simulink model "Dynamic_Formation"  (R2014a)
settings: Solver=ode45  StartTime=0.0  StopTime=800  RelTol=1e-3
settings Model: Creator=asus  LastModifiedBy=asus

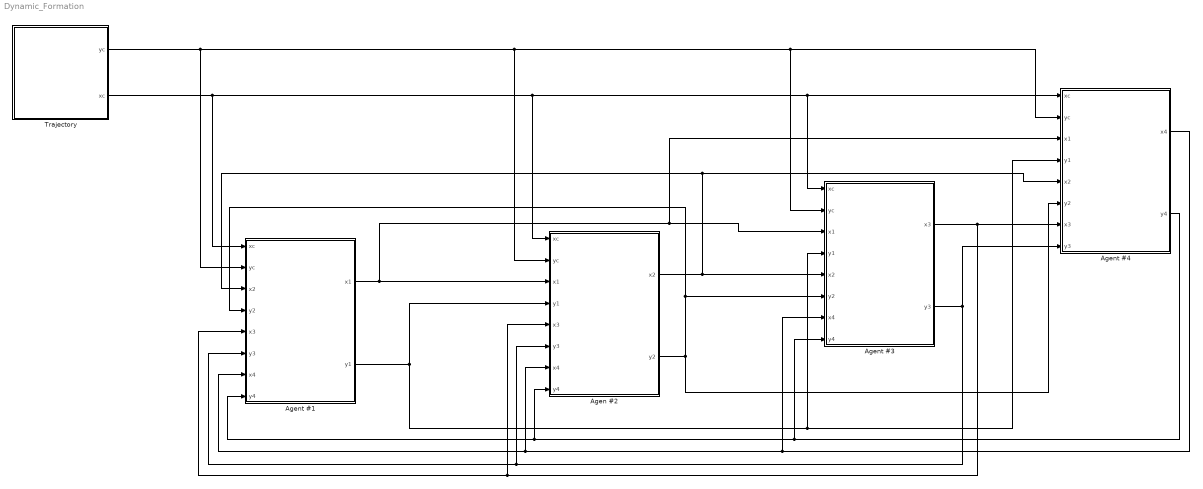
== system Dynamic_Formation ==
  "Agen #2 " : Subsystem
  "Agent #1 " : Subsystem
  Agent #3 : Subsystem
  Agent #4 : Subsystem
  Trajectory : Subsystem
  wires:
  "Agent #1 "/1(x1) -> Agent #4/3(x1), Agent #3/3(x1), "Agen #2 "/3(x1)
  "Agent #1 "/2(y1) -> "Agen #2 "/4(y1), Agent #3/4(y1), Agent #4/4(y1)
  Agent #3/1(x3) -> "Agent #1 "/5(x3), "Agen #2 "/5(x3), Agent #4/7(x3)
  Agent #3/2(y3) -> "Agent #1 "/6(y3), "Agen #2 "/6(y3), Agent #4/8(y3)
  Trajectory/2(xc) -> "Agen #2 "/1(xc), Agent #3/1(xc), Agent #4/1(xc), "Agent #1 "/1(xc)
  Trajectory/1(yc) -> "Agen #2 "/2(yc), Agent #3/2(yc), Agent #4/2(yc), "Agent #1 "/2(yc)
  Agent #4/2(y4) -> "Agent #1 "/8(y4), "Agen #2 "/8(y4), Agent #3/8(y4)
  Agent #4/1(x4) -> "Agent #1 "/7(x4), "Agen #2 "/7(x4), Agent #3/7(x4)
  "Agen #2 "/1(x2) -> "Agent #1 "/3(x2), Agent #4/5(x2), Agent #3/5(x2)
  "Agen #2 "/2(y2) -> Agent #3/6(y2), "Agent #1 "/4(y2), Agent #4/6(y2)

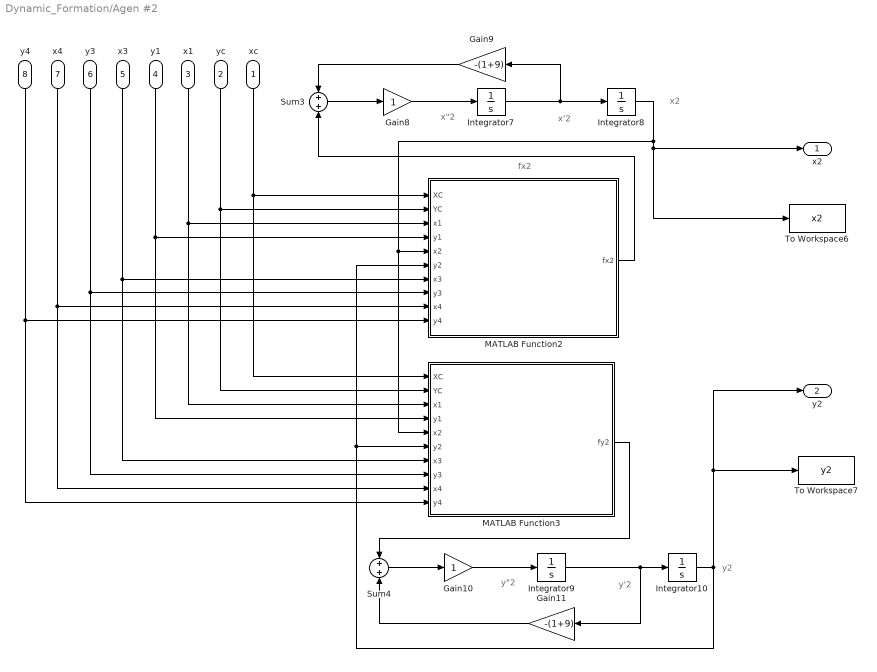
== system Dynamic_Formation/Agen #2  ==
  note: x2
  note: x'2
  note: x"2
  note: fx2
  note: y2
  note: y'2
  note: y"2
  xc : Inport
  yc : Inport  Port=2
  x1 : Inport  Port=3
  y1 : Inport  Port=4
  x3 : Inport  Port=5
  y3 : Inport  Port=6
  x4 : Inport  Port=7
  y4 : Inport  Port=8
  Gain10 : Gain
  Gain11 : Gain  Gain=-(1+9)
  Gain8 : Gain
  Gain9 : Gain  Gain=-(1+9)
  Integrator10 : Integrator  InitialCondition=6
  Integrator7 : Integrator
  Integrator8 : Integrator  InitialCondition=3
  Integrator9 : Integrator
  MATLAB Function2 : MATLAB Function  TreatAsAtomicUnit=on
  MATLAB Function3 : MATLAB Function  TreatAsAtomicUnit=on
  Sum3 : Sum  Inputs=+|+
  Sum4 : Sum  Inputs=+|+
  To Workspace6 : ToWorkspace  VariableName=x2  SampleTime=0.01
  To Workspace7 : ToWorkspace  VariableName=y2  SampleTime=0.01
  x2 : Outport
  y2 : Outport  Port=2
  wires:
  Sum3/1 -> Gain8/1
  Gain8/1 -> Integrator7/1
  Integrator7/1 -> Gain9/1, Integrator8/1
  Gain9/1 -> Sum3/1
  Integrator8/1 -> To Workspace6/1, x2/1, MATLAB Function3/5(x2), MATLAB Function2/5(x2)
  MATLAB Function2/1(fx2) -> Sum3/2
  Sum4/1 -> Gain10/1
  Gain10/1 -> Integrator9/1
  Integrator9/1 -> Gain11/1, Integrator10/1
  Gain11/1 -> Sum4/2
  MATLAB Function3/1(fy2) -> Sum4/1
  Integrator10/1 -> y2/1, To Workspace7/1, MATLAB Function2/6(y2), MATLAB Function3/6(y2)
  xc/1 -> MATLAB Function2/1(XC), MATLAB Function3/1(XC)
  yc/1 -> MATLAB Function2/2(YC), MATLAB Function3/2(YC)
  y1/1 -> MATLAB Function2/4(y1), MATLAB Function3/4(y1)
  x1/1 -> MATLAB Function2/3(x1), MATLAB Function3/3(x1)
  x3/1 -> MATLAB Function2/7(x3), MATLAB Function3/7(x3)
  y3/1 -> MATLAB Function2/8(y3), MATLAB Function3/8(y3)
  x4/1 -> MATLAB Function2/9(x4), MATLAB Function3/9(x4)
  y4/1 -> MATLAB Function2/10(y4), MATLAB Function3/10(y4)

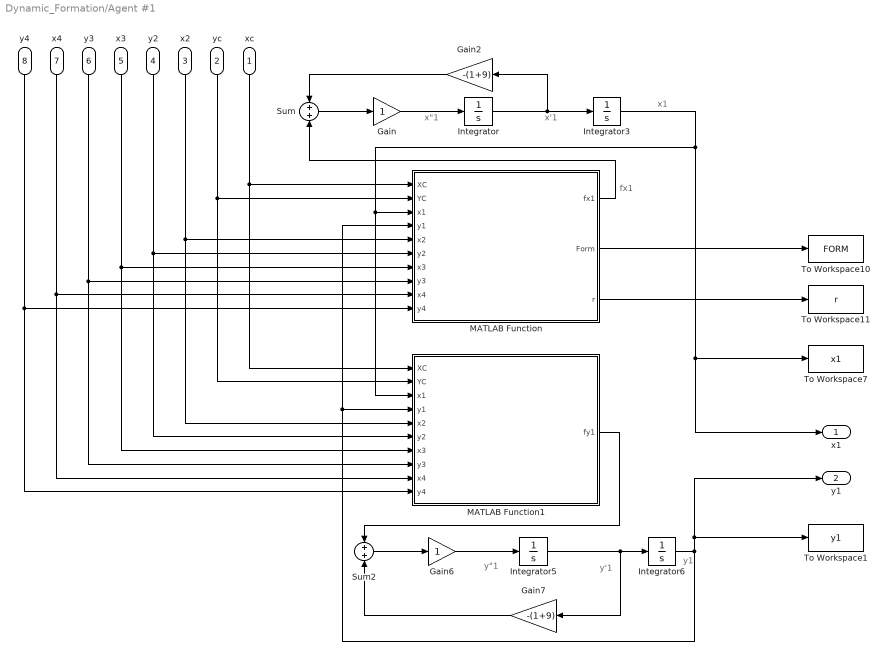
== system Dynamic_Formation/Agent #1  ==
  note: x1
  note: x'1
  note: x"1
  note: fx1
  note: y1
  note: y'1
  note: y"1
  xc : Inport
  yc : Inport  Port=2
  x2 : Inport  Port=3
  y2 : Inport  Port=4
  x3 : Inport  Port=5
  y3 : Inport  Port=6
  x4 : Inport  Port=7
  y4 : Inport  Port=8
  Gain : Gain
  Gain2 : Gain  Gain=-(1+9)
  Gain6 : Gain
  Gain7 : Gain  Gain=-(1+9)
  Integrator : Integrator
  Integrator3 : Integrator  InitialCondition=-1
  Integrator5 : Integrator
  Integrator6 : Integrator  InitialCondition=2
  MATLAB Function : MATLAB Function  TreatAsAtomicUnit=on
  MATLAB Function1 : MATLAB Function  TreatAsAtomicUnit=on
  Sum : Sum  Inputs=+|+
  Sum2 : Sum  Inputs=+|+
  To Workspace1 : ToWorkspace  VariableName=y1  SampleTime=0.01
  To Workspace10 : ToWorkspace  VariableName=FORM  SampleTime=0.01
  To Workspace11 : ToWorkspace  VariableName=r  SampleTime=1
  To Workspace7 : ToWorkspace  VariableName=x1  SampleTime=0.01
  x1 : Outport
  y1 : Outport  Port=2
  wires:
  Sum/1 -> Gain/1
  Gain/1 -> Integrator/1
  Integrator/1 -> Gain2/1, Integrator3/1
  Gain2/1 -> Sum/1
  Sum2/1 -> Gain6/1
  Gain6/1 -> Integrator5/1
  Integrator5/1 -> Gain7/1, Integrator6/1
  Gain7/1 -> Sum2/2
  MATLAB Function1/1(fy1) -> Sum2/1
  Integrator6/1 -> MATLAB Function/4(y1), MATLAB Function1/4(y1), To Workspace1/1, y1/1
  MATLAB Function/1(fx1) -> Sum/2
  MATLAB Function/2(Form) -> To Workspace10/1
  MATLAB Function/3(r) -> To Workspace11/1
  Integrator3/1 -> MATLAB Function1/3(x1), MATLAB Function/3(x1), To Workspace7/1, x1/1
  xc/1 -> MATLAB Function/1(XC), MATLAB Function1/1(XC)
  yc/1 -> MATLAB Function/2(YC), MATLAB Function1/2(YC)
  x2/1 -> MATLAB Function/5(x2), MATLAB Function1/5(x2)
  y2/1 -> MATLAB Function/6(y2), MATLAB Function1/6(y2)
  x3/1 -> MATLAB Function/7(x3), MATLAB Function1/7(x3)
  y3/1 -> MATLAB Function/8(y3), MATLAB Function1/8(y3)
  x4/1 -> MATLAB Function/9(x4), MATLAB Function1/9(x4)
  y4/1 -> MATLAB Function/10(y4), MATLAB Function1/10(y4)

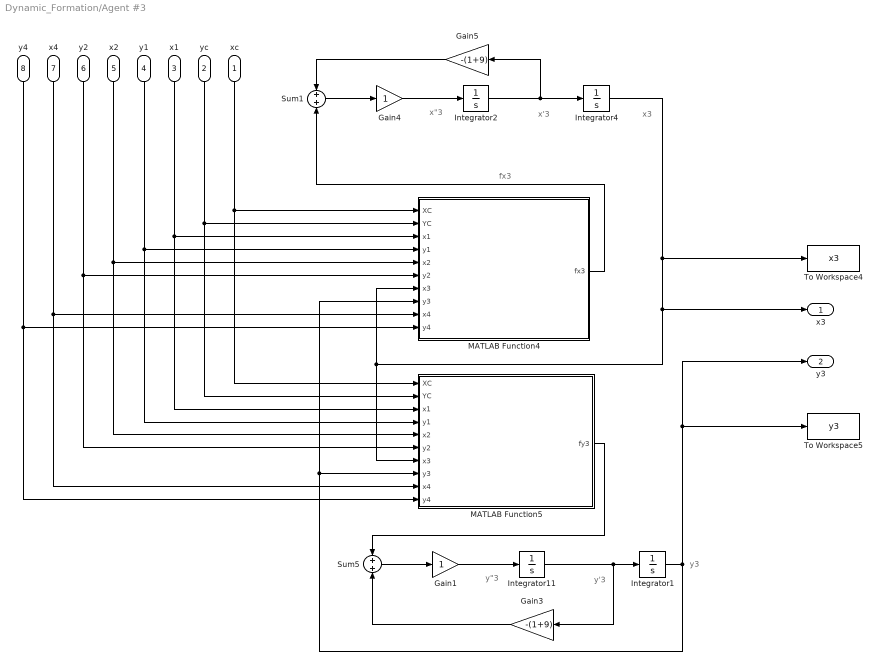
== system Dynamic_Formation/Agent #3 ==
  note: x3
  note: x'3
  note: x"3
  note: fx3
  note: y3
  note: y'3
  note: y"3
  xc : Inport
  yc : Inport  Port=2
  x1 : Inport  Port=3
  y1 : Inport  Port=4
  x2 : Inport  Port=5
  y2 : Inport  Port=6
  x4 : Inport  Port=7
  y4 : Inport  Port=8
  Gain1 : Gain
  Gain3 : Gain  Gain=-(1+9)
  Gain4 : Gain
  Gain5 : Gain  Gain=-(1+9)
  Integrator1 : Integrator  InitialCondition=-1
  Integrator11 : Integrator
  Integrator2 : Integrator
  Integrator4 : Integrator  InitialCondition=3
  MATLAB Function4 : MATLAB Function  TreatAsAtomicUnit=on
  MATLAB Function5 : MATLAB Function  TreatAsAtomicUnit=on
  Sum1 : Sum  Inputs=+|+
  Sum5 : Sum  Inputs=+|+
  To Workspace4 : ToWorkspace  VariableName=x3  SampleTime=0.01
  To Workspace5 : ToWorkspace  VariableName=y3  SampleTime=0.01
  x3 : Outport
  y3 : Outport  Port=2
  wires:
  Sum1/1 -> Gain4/1
  Gain4/1 -> Integrator2/1
  Integrator2/1 -> Gain5/1, Integrator4/1
  Gain5/1 -> Sum1/1
  MATLAB Function4/1(fx3) -> Sum1/2
  Sum5/1 -> Gain1/1
  Gain1/1 -> Integrator11/1
  Integrator11/1 -> Gain3/1, Integrator1/1
  Gain3/1 -> Sum5/2
  MATLAB Function5/1(fy3) -> Sum5/1
  Integrator1/1 -> MATLAB Function5/8(y3), MATLAB Function4/8(y3), To Workspace5/1, y3/1
  Integrator4/1 -> x3/1, MATLAB Function5/7(x3), MATLAB Function4/7(x3), To Workspace4/1
  xc/1 -> MATLAB Function4/1(XC), MATLAB Function5/1(XC)
  yc/1 -> MATLAB Function5/2(YC), MATLAB Function4/2(YC)
  x1/1 -> MATLAB Function4/3(x1), MATLAB Function5/3(x1)
  y1/1 -> MATLAB Function4/4(y1), MATLAB Function5/4(y1)
  x2/1 -> MATLAB Function4/5(x2), MATLAB Function5/5(x2)
  y2/1 -> MATLAB Function4/6(y2), MATLAB Function5/6(y2)
  x4/1 -> MATLAB Function4/9(x4), MATLAB Function5/9(x4)
  y4/1 -> MATLAB Function4/10(y4), MATLAB Function5/10(y4)

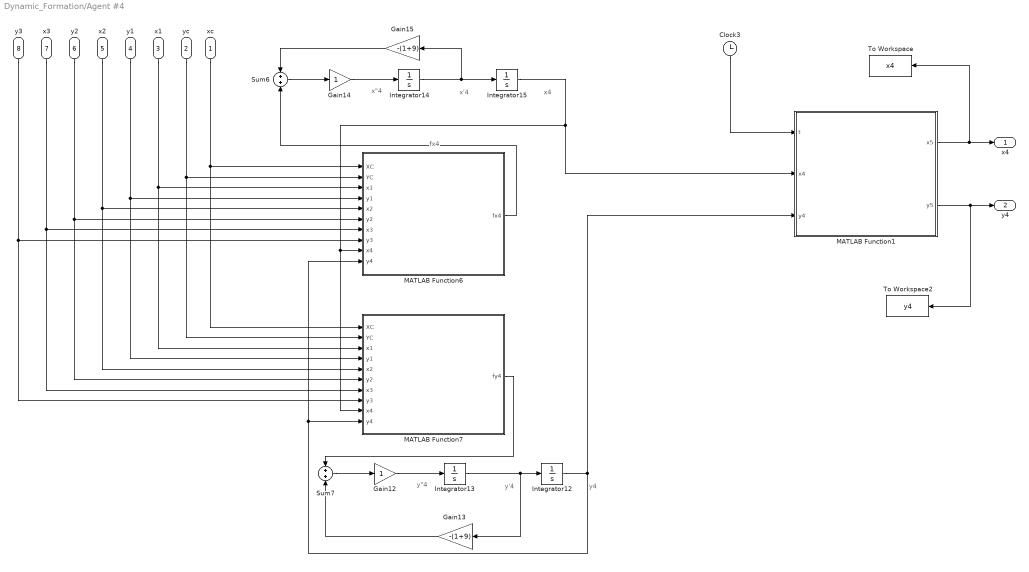
== system Dynamic_Formation/Agent #4 ==
  note: x4
  note: x'4
  note: x"4
  note: fx4
  note: y4
  note: y'4
  note: y"4
  xc : Inport
  yc : Inport  Port=2
  x1 : Inport  Port=3
  y1 : Inport  Port=4
  x2 : Inport  Port=5
  y2 : Inport  Port=6
  x3 : Inport  Port=7
  y3 : Inport  Port=8
  Clock3 : Clock
  Gain12 : Gain
  Gain13 : Gain  Gain=-(1+9)
  Gain14 : Gain
  Gain15 : Gain  Gain=-(1+9)
  Integrator12 : Integrator  InitialCondition=-4
  Integrator13 : Integrator
  Integrator14 : Integrator
  Integrator15 : Integrator  InitialCondition=-4
  MATLAB Function1 : MATLAB Function  TreatAsAtomicUnit=on
  MATLAB Function6 : MATLAB Function  TreatAsAtomicUnit=on
  MATLAB Function7 : MATLAB Function  TreatAsAtomicUnit=on
  Sum6 : Sum  Inputs=+|+
  Sum7 : Sum  Inputs=+|+
  To Workspace : ToWorkspace  VariableName=x4  SampleTime=0.01
  To Workspace2 : ToWorkspace  VariableName=y4  SampleTime=0.01
  x4 : Outport
  y4 : Outport  Port=2
  wires:
  Sum6/1 -> Gain14/1
  Gain14/1 -> Integrator14/1
  Integrator14/1 -> Gain15/1, Integrator15/1
  Gain15/1 -> Sum6/1
  Integrator15/1 -> MATLAB Function1/2(x4), MATLAB Function7/9(x4), MATLAB Function6/9(x4)
  MATLAB Function6/1(fx4) -> Sum6/2
  Sum7/1 -> Gain12/1
  Gain12/1 -> Integrator13/1
  Integrator13/1 -> Gain13/1, Integrator12/1
  Gain13/1 -> Sum7/2
  MATLAB Function7/1(fy4) -> Sum7/1
  Integrator12/1 -> MATLAB Function1/3(y4), MATLAB Function6/10(y4), MATLAB Function7/10(y4)
  Clock3/1 -> MATLAB Function1/1(t)
  xc/1 -> MATLAB Function6/1(XC), MATLAB Function7/1(XC)
  yc/1 -> MATLAB Function6/2(YC), MATLAB Function7/2(YC)
  x1/1 -> MATLAB Function6/3(x1), MATLAB Function7/3(x1)
  y1/1 -> MATLAB Function6/4(y1), MATLAB Function7/4(y1)
  x2/1 -> MATLAB Function6/5(x2), MATLAB Function7/5(x2)
  y2/1 -> MATLAB Function6/6(y2), MATLAB Function7/6(y2)
  x3/1 -> MATLAB Function6/7(x3), MATLAB Function7/7(x3)
  y3/1 -> MATLAB Function6/8(y3), MATLAB Function7/8(y3)
  MATLAB Function1/1(x5) -> To Workspace/1, x4/1
  MATLAB Function1/2(y5) -> To Workspace2/1, y4/1

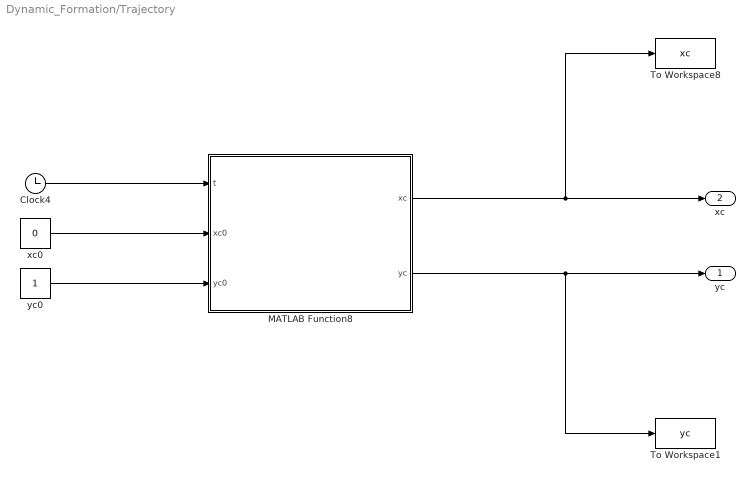
== system Dynamic_Formation/Trajectory ==
  Clock4 : Clock
  MATLAB Function8 : MATLAB Function  TreatAsAtomicUnit=on
  To Workspace1 : ToWorkspace  VariableName=yc  SampleTime=0.01
  To Workspace8 : ToWorkspace  VariableName=xc  SampleTime=0.01
  xc0 : Constant  Value=0
  yc0 : Constant
  yc : Outport
  xc : Outport  Port=2
  wires:
  xc0/1 -> MATLAB Function8/2(xc0)
  yc0/1 -> MATLAB Function8/3(yc0)
  Clock4/1 -> MATLAB Function8/1(t)
  MATLAB Function8/1(xc) -> To Workspace8/1, xc/1
  MATLAB Function8/2(yc) -> To Workspace1/1, yc/1

== matlab function Dynamic_Formation/Agent #1 /MATLAB Function1 ==
  data: XC input; YC input; fy1 output; x1 input; y1 input; x2 input; y2 input; x3 input; y3 input; x4 input; y4 input
function fy1 = fy1(XC,YC,x1,y1,x2,y2,x3,y3,x4,y4)
%#codegen
% Agent N#1
%xc = sin(t);
%yc = t;
%xc = XC;            % X-Center.
%yc = YC;            % Y-Center.
al = 3;             % Radius.
x = [x1 x2 x3 x4];      
y = [y1 y2 y3 y4];     
M = 1;              % Mass.
B = 1;              % Damper.
kd = 9;             % Overshoot Controlling Coefficient.
ks = 1;
q = 10;     % Charges.
kr = 0.15;
N = 4;              % Number od Agents.

r2 = zeros(N,N);
costet = zeros(N,N);
sintet = zeros(N,N);
Prx = zeros(N);
Pry = zeros(N);

fx = zeros(N);
fy = zeros(N);
Fx = zeros(N);
Fy = zeros(N);


d1 = sqrt(((x(1)-XC)^2)+((y(1)-YC)^2));
d2 = sqrt(((x(2)-XC)^2)+((y(2)-YC)^2));
d3 = sqrt(((x(3)-XC)^2)+((y(3)-YC)^2));
d4 = sqrt(((x(4)-XC)^2)+((y(4)-YC)^2));
    
m1 = d2-d1;
m2 = d3-d2;
m3 = d4-d3;
    
    if m1<0.00001
        if m2<0.00001
            if m3<0.00001
                Form = 1;
            else
                Form = 0;
            end
        else
            Form = 0;
        end
    else 
        Form = 0;
    end

    
%if Form==0
    xc = XC;            % X-Center.
    yc = YC;            % Y-Center.



for k=1:N
    
    for i=1:N
      Pr = 0;
      r2(k,i) = ((x(i)-x(k))^2)+((y(i)-y(k))^2);
    
      if i==k
         Prx(k) = Prx(k) + 0;
         Pry(k) = Pry(k) + 0;
      else
         costet(k,i) = (x(k)-x(i))/sqrt(r2(k,i));
         sintet(k,i) = (y(k)-y(i))/sqrt(r2(k,i));
         Prx(k) = Prx(k) + (q*q/r2(k,i))*costet(k,i);
         Pry(k) = Pry(k) + (q*q/r2(k,i))*sintet(k,i);
        
      end
    end

    Fx(k) = kr*Prx(k);
    Fy(k) = kr*Pry(k);
                        
    fx(k) = Fx(k)-ks*((x(k)-xc)*(((x(k)-xc)^2)+((y(k)-yc)^2)-al^2));
    fy(k) = Fy(k)-ks*((y(k)-yc)*(((x(k)-xc)^2)+((y(k)-yc)^2)-al^2));

end

fy1 = fy(1);

end

== matlab function Dynamic_Formation/Agent #1 /MATLAB Function ==
  data: XC input; YC input; fx1 output; x1 input; y1 input; x2 input; y2 input; x3 input; y3 input; x4 input; y4 input; Form output; r output
function [fx1,Form,r] = fx1(XC,YC,x1,y1,x2,y2,x3,y3,x4,y4)
%#codegen
% Agent N#1

xc = XC;            % X-Center.
yc = YC;            % Y-Center.
%xc = 0;            % X-Center.
%yc = 0;            % Y-Center.
al = 3;             % Radius.
x = [x1 x2 x3 x4];  % x vector.    
y = [y1 y2 y3 y4];  % y vector.   
M = 1;              % Mass.
B = 1;              % Damper.
kd = 9;             % Overshoot Controlling Coefficient.
ks = 1;
q = 10;             % Charges.
kr = 0.15;
N = 4;              % Number od Agents.
H = 0;

r2 = zeros(N,N);
costet = zeros(N,N);
sintet = zeros(N,N);
Prx = zeros(N);
Pry = zeros(N);
fx = zeros(N);
fy = zeros(N);
Fx = zeros(N);
Fy = zeros(N);

d1 = sqrt(((x(1)-XC)^2)+((y(1)-YC)^2));
d2 = sqrt(((x(2)-XC)^2)+((y(2)-YC)^2));
d3 = sqrt(((x(3)-XC)^2)+((y(3)-YC)^2));
d4 = sqrt(((x(4)-XC)^2)+((y(4)-YC)^2));

m1 = d2-d1;
m2 = d3-d2;
m3 = d4-d3;
    
    if m1<0.00001
        if m2<0.00001
            if m3<0.00001
                Form = 1;
            else
                Form = 0;
            end
        else
            Form = 0;
        end
    else 
        Form = 0;
    end


    
    for k=1:N
    
        for i=1:N
            Pr = 0;
            r2(k,i) = ((x(i)-x(k))^2)+((y(i)-y(k))^2);
    
         if i==k
             Prx(k) = Prx(k) + 0;
            Pry(k) = Pry(k) + 0;
         else
            costet(k,i) = (x(k)-x(i))/sqrt(r2(k,i));
            sintet(k,i) = (y(k)-y(i))/sqrt(r2(k,i));
            Prx(k) = Prx(k) + (q*q/r2(k,i))*costet(k,i);
            Pry(k) = Pry(k) + (q*q/r2(k,i))*sintet(k,i);
        
         end
        end

     Fx(k) = kr*Prx(k);
     Fy(k) = kr*Pry(k);
                        
     fx(k) = Fx(k)-ks*((x(k)-xc)*(((x(k)-xc)^2)+((y(k)-yc)^2)-al^2));
     fy(k) = Fy(k)-ks*((y(k)-yc)*(((x(k)-xc)^2)+((y(k)-yc)^2)-al^2));

    end

    fx1 = fx(1);
    r=r2;
    

   
    
    
    
    
    
    
    
    
    
    
    


end

== matlab function Dynamic_Formation/Agen #2 /MATLAB Function2 ==
  data: XC input; YC input; fx2 output; x1 input; y1 input; x2 input; y2 input; x3 input; y3 input; x4 input; y4 input
function fx2 = fx2(XC,YC,x1,y1,x2,y2,x3,y3,x4,y4)
%#codegen
% Agent N#1
%xc = XC;            % X-Center.
%yc = YC;            % Y-Center.
%xc = 0;             % X-Center.
%yc = 0;             % Y-Center.
al = 3;             % Radius.
x = [x1 x2 x3 x4];      
y = [y1 y2 y3 y4];     
M = 1;              % Mass.
B = 1;              % Damper.
kd = 9;             % Overshoot Controlling Coefficient.
ks = 1;
q = 10;     % Charges.
kr = 0.15;
N = 4;              % Number od Agents.

r2 = zeros(N,N);
costet = zeros(N,N);
sintet = zeros(N,N);
Prx = zeros(N);
Pry = zeros(N);

fx = zeros(N);
fy = zeros(N);
Fx = zeros(N);
Fy = zeros(N);

d1 = sqrt(((x(1)-XC)^2)+((y(1)-YC)^2));
d2 = sqrt(((x(2)-XC)^2)+((y(2)-YC)^2));
d3 = sqrt(((x(3)-XC)^2)+((y(3)-YC)^2));
d4 = sqrt(((x(4)-XC)^2)+((y(4)-YC)^2));
    
m1 = d2-d1;
m2 = d3-d2;
m3 = d4-d3;
    
    if m1<0.00001
        if m2<0.00001
            if m3<0.00001
                Form = 1;
            else
                Form = 0;
            end
        else
            Form = 0;
        end
    else 
        Form = 0;
    end

    
    xc = XC;            % X-Center.
    yc = YC;            % Y-Center.




for k=1:N
    
    for i=1:N
      Pr = 0;
      r2(k,i) = ((x(i)-x(k))^2)+((y(i)-y(k))^2);
    
      if i==k
         Prx(k) = Prx(k) + 0;
         Pry(k) = Pry(k) + 0;
      else
         costet(k,i) = (x(k)-x(i))/sqrt(r2(k,i));
         sintet(k,i) = (y(k)-y(i))/sqrt(r2(k,i));
         Prx(k) = Prx(k) + (q*q/r2(k,i))*costet(k,i);
         Pry(k) = Pry(k) + (q*q/r2(k,i))*sintet(k,i);
        
      end
    end

    Fx(k) = kr*Prx(k);
    Fy(k) = kr*Pry(k);
                        
    fx(k) = Fx(k)-ks*((x(k)-xc)*(((x(k)-xc)^2)+((y(k)-yc)^2)-al^2));
    fy(k) = Fy(k)-ks*((y(k)-yc)*(((x(k)-xc)^2)+((y(k)-yc)^2)-al^2));

end

fx2 = fx(2);


end

== matlab function Dynamic_Formation/Agen #2 /MATLAB Function3 ==
  data: XC input; YC input; fy2 output; x1 input; y1 input; x2 input; y2 input; x3 input; y3 input; x4 input; y4 input
function fy2 = fy2(XC,YC,x1,y1,x2,y2,x3,y3,x4,y4)
%#codegen
% Agent N#1
%yc = YC;            % Y-Center.
al = 3;             % Radius.
x = [x1 x2 x3 x4];      
y = [y1 y2 y3 y4];     
M = 1;              % Mass.
B = 1;              % Damper.
kd = 9;             % Overshoot Controlling Coefficient.
ks = 1;
q = 10;     % Charges.
kr = 0.15;
N = 4;              % Number od Agents.

r2 = zeros(N,N);
costet = zeros(N,N);
sintet = zeros(N,N);
Prx = zeros(N);
Pry = zeros(N);

fx = zeros(N);
fy = zeros(N);
Fx = zeros(N);
Fy = zeros(N);

d1 = sqrt(((x(1)-XC)^2)+((y(1)-YC)^2));
d2 = sqrt(((x(2)-XC)^2)+((y(2)-YC)^2));
d3 = sqrt(((x(3)-XC)^2)+((y(3)-YC)^2));
d4 = sqrt(((x(4)-XC)^2)+((y(4)-YC)^2));
    
m1 = d2-d1;
m2 = d3-d2;
m3 = d4-d3;
    
    if m1<0.00001
        if m2<0.00001
            if m3<0.00001
                Form = 1;
            else
                Form = 0;
            end
        else
            Form = 0;
        end
    else 
        Form = 0;
    end


    
    xc = XC;            % X-Center.
    yc = YC;            % Y-Center.




for k=1:N
    
    for i=1:N
      Pr = 0;
      r2(k,i) = ((x(i)-x(k))^2)+((y(i)-y(k))^2);
    
      if i==k
         Prx(k) = Prx(k) + 0;
         Pry(k) = Pry(k) + 0;
      else
         costet(k,i) = (x(k)-x(i))/sqrt(r2(k,i));
         sintet(k,i) = (y(k)-y(i))/sqrt(r2(k,i));
         Prx(k) = Prx(k) + (q*q/r2(k,i))*costet(k,i);
         Pry(k) = Pry(k) + (q*q/r2(k,i))*sintet(k,i);
        
      end
    end

    Fx(k) = kr*Prx(k);
    Fy(k) = kr*Pry(k);
                        
    fx(k) = Fx(k)-ks*((x(k)-xc)*(((x(k)-xc)^2)+((y(k)-yc)^2)-al^2));
    fy(k) = Fy(k)-ks*((y(k)-yc)*(((x(k)-xc)^2)+((y(k)-yc)^2)-al^2));

end

fy2 = fy(2);


end

== matlab function Dynamic_Formation/Agent #3/MATLAB Function4 ==
  data: XC input; YC input; fx3 output; x1 input; y1 input; x2 input; y2 input; x3 input; y3 input; x4 input; y4 input
function fx3 = fx3(XC,YC,x1,y1,x2,y2,x3,y3,x4,y4)
%#codegen
% Agent N#1
al = 3;             % Radius.
x = [x1 x2 x3 x4];      
y = [y1 y2 y3 y4];     
M = 1;              % Mass.
B = 1;              % Damper.
kd = 9;             % Overshoot Controlling Coefficient.
ks = 1;
q = 10;     % Charges.
kr = 0.15;
N = 4;              % Number od Agents.

r2 = zeros(N,N);
costet = zeros(N,N);
sintet = zeros(N,N);
Prx = zeros(N);
Pry = zeros(N);

fx = zeros(N);
fy = zeros(N);
Fx = zeros(N);
Fy = zeros(N);


Form = 0;
d1 = sqrt(((x(1)-XC)^2)+((y(1)-YC)^2));
d2 = sqrt(((x(2)-XC)^2)+((y(2)-YC)^2));
d3 = sqrt(((x(3)-XC)^2)+((y(3)-YC)^2));
d4 = sqrt(((x(4)-XC)^2)+((y(4)-YC)^2));
    
m1 = d2-d1;
m2 = d3-d2;
m3 = d4-d3;
    
    if m1<0.00001
        if m2<0.00001
            if m3<0.00001
                Form = 1;
            end
        end
    end

    
    xc = XC;            % X-Center.
    yc = YC;            % Y-Center.




for k=1:N
    
    for i=1:N
      Pr = 0;
      r2(k,i) = ((x(i)-x(k))^2)+((y(i)-y(k))^2);
    
      if i==k
         Prx(k) = Prx(k) + 0;
         Pry(k) = Pry(k) + 0;
      else
         costet(k,i) = (x(k)-x(i))/sqrt(r2(k,i));
         sintet(k,i) = (y(k)-y(i))/sqrt(r2(k,i));
         Prx(k) = Prx(k) + (q*q/r2(k,i))*costet(k,i);
         Pry(k) = Pry(k) + (q*q/r2(k,i))*sintet(k,i);
        
      end
    end

    Fx(k) = kr*Prx(k);
    Fy(k) = kr*Pry(k);
                        
    fx(k) = Fx(k)-ks*((x(k)-xc)*(((x(k)-xc)^2)+((y(k)-yc)^2)-al^2));
    fy(k) = Fy(k)-ks*((y(k)-yc)*(((x(k)-xc)^2)+((y(k)-yc)^2)-al^2));

end

fx3 = fx(3);


end

== matlab function Dynamic_Formation/Agent #3/MATLAB Function5 ==
  data: XC input; YC input; fy3 output; x1 input; y1 input; x2 input; y2 input; x3 input; y3 input; x4 input; y4 input
function fy3 = fy3(XC,YC,x1,y1,x2,y2,x3,y3,x4,y4)
%#codegen
al = 3;             % Radius.
x = [x1 x2 x3 x4];      
y = [y1 y2 y3 y4];     
M = 1;              % Mass.
B = 1;              % Damper.
kd = 9;             % Overshoot Controlling Coefficient.
ks = 1;
q = 10;     % Charges.
kr = 0.15;
N = 4;              % Number od Agents.

r2 = zeros(N,N);
costet = zeros(N,N);
sintet = zeros(N,N);
Prx = zeros(N);
Pry = zeros(N);

fx = zeros(N);
fy = zeros(N);
Fx = zeros(N);
Fy = zeros(N);

Form = 0;
d1 = sqrt(((x(1)-XC)^2)+((y(1)-YC)^2));
d2 = sqrt(((x(2)-XC)^2)+((y(2)-YC)^2));
d3 = sqrt(((x(3)-XC)^2)+((y(3)-YC)^2));
d4 = sqrt(((x(4)-XC)^2)+((y(4)-YC)^2));
    
m1 = d2-d1;
m2 = d3-d2;
m3 = d4-d3;
    
    if m1<0.00001
        if m2<0.00001
            if m3<0.00001
                Form = 1;
            end
        end
    end

    
%if Form==0
    xc = XC;            % X-Center.
    yc = YC;            % Y-Center.



for k=1:N
    
    for i=1:N
      Pr = 0;
      r2(k,i) = ((x(i)-x(k))^2)+((y(i)-y(k))^2);
    
      if i==k
         Prx(k) = Prx(k) + 0;
         Pry(k) = Pry(k) + 0;
      else
         costet(k,i) = (x(k)-x(i))/sqrt(r2(k,i));
         sintet(k,i) = (y(k)-y(i))/sqrt(r2(k,i));
         Prx(k) = Prx(k) + (q*q/r2(k,i))*costet(k,i);
         Pry(k) = Pry(k) + (q*q/r2(k,i))*sintet(k,i);
        
      end
    end

    Fx(k) = kr*Prx(k);
    Fy(k) = kr*Pry(k);
                        
    fx(k) = Fx(k)-ks*((x(k)-xc)*(((x(k)-xc)^2)+((y(k)-yc)^2)-al^2));
    fy(k) = Fy(k)-ks*((y(k)-yc)*(((x(k)-xc)^2)+((y(k)-yc)^2)-al^2));

end

fy3 = fy(3);


end

== matlab function Dynamic_Formation/Agent #4/MATLAB Function6 ==
  data: XC input; YC input; fx4 output; x1 input; y1 input; x2 input; y2 input; x3 input; y3 input; x4 input; y4 input
function fx4 = fx4(XC,YC,x1,y1,x2,y2,x3,y3,x4,y4)
%#codegen
al = 3;             % Radius.
x = [x1 x2 x3 x4];      
y = [y1 y2 y3 y4];     
M = 1;              % Mass.
B = 1;              % Damper.
kd = 9;             % Overshoot Controlling Coefficient.
ks = 1;
q = 10;     % Charges.
kr = 0.15;
N = 4;              % Number od Agents.

r2 = zeros(N,N);
costet = zeros(N,N);
sintet = zeros(N,N);
Prx = zeros(N);
Pry = zeros(N);

fx = zeros(N);
fy = zeros(N);
Fx = zeros(N);
Fy = zeros(N);

Form = 0;
d1 = sqrt(((x(1)-XC)^2)+((y(1)-YC)^2));
d2 = sqrt(((x(2)-XC)^2)+((y(2)-YC)^2));
d3 = sqrt(((x(3)-XC)^2)+((y(3)-YC)^2));
d4 = sqrt(((x(4)-XC)^2)+((y(4)-YC)^2));
    
m1 = d2-d1;
m2 = d3-d2;
m3 = d4-d3;
    
    if m1<0.00001
        if m2<0.00001
            if m3<0.00001
                Form = 1;
            end
        end
    end

    
    xc = XC;            % X-Center.
    yc = YC;          


for k=1:N
    
    for i=1:N
      Pr = 0;
      r2(k,i) = ((x(i)-x(k))^2)+((y(i)-y(k))^2);
    
      if i==k
         Prx(k) = Prx(k) + 0;
         Pry(k) = Pry(k) + 0;
      else
         costet(k,i) = (x(k)-x(i))/sqrt(r2(k,i));
         sintet(k,i) = (y(k)-y(i))/sqrt(r2(k,i));
         Prx(k) = Prx(k) + (q*q/r2(k,i))*costet(k,i);
         Pry(k) = Pry(k) + (q*q/r2(k,i))*sintet(k,i);
        
      end
    end

    Fx(k) = kr*Prx(k);
    Fy(k) = kr*Pry(k);
                        
    fx(k) = Fx(k)-ks*((x(k)-xc)*(((x(k)-xc)^2)+((y(k)-yc)^2)-al^2));
    fy(k) = Fy(k)-ks*((y(k)-yc)*(((x(k)-xc)^2)+((y(k)-yc)^2)-al^2));

end

fx4 = fx(4);


end

== matlab function Dynamic_Formation/Agent #4/MATLAB Function7 ==
  data: XC input; YC input; fy4 output; x1 input; y1 input; x2 input; y2 input; x3 input; y3 input; x4 input; y4 input
function fy4 = fy4(XC,YC,x1,y1,x2,y2,x3,y3,x4,y4)
%#codegen
al = 3;             % Radius.
x = [x1 x2 x3 x4];      
y = [y1 y2 y3 y4];     
M = 1;              % Mass.
B = 1;              % Damper.
kd = 9;             % Overshoot Controlling Coefficient.
ks = 1;
q = 10;             % Charges.
kr = 0.15;
N = 4;              % Number of Agents.

r2 = zeros(N,N);
costet = zeros(N,N);
sintet = zeros(N,N);
Prx = zeros(N);
Pry = zeros(N);

fx = zeros(N);
fy = zeros(N);
Fx = zeros(N);
Fy = zeros(N);

Form = 0;
d1 = sqrt(((x(1)-XC)^2)+((y(1)-YC)^2));
d2 = sqrt(((x(2)-XC)^2)+((y(2)-YC)^2));
d3 = sqrt(((x(3)-XC)^2)+((y(3)-YC)^2));
d4 = sqrt(((x(4)-XC)^2)+((y(4)-YC)^2));
    
m1 = d2-d1;
m2 = d3-d2;
m3 = d4-d3;
    
    if m1<0.00001
        if m2<0.00001
            if m3<0.00001
                Form = 1;
            end
        end
    end

    
    xc = XC;            % X-Center.
    yc = YC;            % Y-Center.
 


for k=1:N
    
    for i=1:N
      Pr = 0;
      r2(k,i) = ((x(i)-x(k))^2)+((y(i)-y(k))^2);
    
      if i==k
         Prx(k) = Prx(k) + 0;
         Pry(k) = Pry(k) + 0;
      else
         costet(k,i) = (x(k)-x(i))/sqrt(r2(k,i));
         sintet(k,i) = (y(k)-y(i))/sqrt(r2(k,i));
         Prx(k) = Prx(k) + (q*q/r2(k,i))*costet(k,i);
         Pry(k) = Pry(k) + (q*q/r2(k,i))*sintet(k,i);
        
      end
    end

    Fx(k) = kr*Prx(k);
    Fy(k) = kr*Pry(k);
                        
    fx(k) = Fx(k)-ks*((x(k)-xc)*(((x(k)-xc)^2)+((y(k)-yc)^2)-al^2));
    fy(k) = Fy(k)-ks*((y(k)-yc)*(((x(k)-xc)^2)+((y(k)-yc)^2)-al^2));

end

fy4 = fy(4);


end

== matlab function Dynamic_Formation/Trajectory/MATLAB Function8 ==
  data: t input; xc0 input; yc0 input; xc output; yc output
function [xc,yc] = trj(t,xc0,yc0)
%#codegen
    xc = xc0;
    yc = yc0;
u = 4*pi/800;
g = 0:u:4*pi;

if t<151
    xc = xc0;
    yc = yc0;
else 
    p0 = (t-150)/50;       % Every 50 sec.
    p1 = ceil(p0);          % Coefficient.
    xc = p1;                 % Expanding the trajectory.
    yc = 2*sin(13*pi*g(p1));
end







end

== matlab function Dynamic_Formation/Agent #4/MATLAB Function1 ==
  data: t input; x5 output; x4 input; y4 input; y5 output
function [x5,y5] = rpb(t,x4,y4)
%#codegen
% A function for elemination of Agent #4 in tiime=400s.

if t<400000
    x5 = x4;
    y5 = y4;

else
    x5 = 99999900000000000000000;
    y5 = 99999900000000000000000;
end

end
